simulink model "Furnace"  (R2020a)
settings: Solver=ode15s  StartTime=0  StopTime=27000  FixedStep=0.1  MaxStep=20  MinStep=1e-13  RelTol=1e-08  AbsTol=1e-09
undefined symbols (not defined in the file): agnostic_lqe_params, cont_reg, disturbance_type, F_aI_pid, F_aII_pid, input_type, k, lqe_params, LQR_params, LQRAgnostic_params, MPC_type, MPCDiscrete_function_parameters, MPCDiscreteAgnostic_function_parameters, MPCDiscreteDiffIntegralAgnostic_function_parameters, original_LQR_params, output_type, reg, single_butter_ss
libraries: simulink x35, cstblocks x10, mpclib x3
(part 8 of 8)

== matlab function Furnace/Deprecated, slow loop/Contineous Summer student feedback (Not finished)/Controller/Input  selector2 ==
  data: constant input; signal output; experimental input; controlled input; input_type input
function signal = ChooseSignal(constant, experimental, controlled, input_type)
    switch(input_type)
        case InputType.Experimental
            signal = experimental;
        case InputType.Controlled
            signal = controlled;
        otherwise
            signal = constant;
    end
end

== matlab function Furnace/Deprecated, slow loop/Contineous Summer student feedback (Not finished)/Controller/Input  selector3 ==
  data: constant input; signal output; experimental input; controlled input; input_type input
function signal = ChooseSignal(constant, experimental, controlled, input_type)
    switch(input_type)
        case InputType.Experimental
            signal = experimental;
        case InputType.Controlled
            signal = controlled;
        otherwise
            signal = constant;
    end
end

== matlab function Furnace/Deprecated, slow loop/Contineous Summer student feedback (Not finished)/Controller/Input  selector4 ==
  data: constant input; signal output; experimental input; controlled input; input_type input
function signal = ChooseSignal(constant, experimental, controlled, input_type)
    switch(input_type)
        case InputType.Experimental
            signal = experimental;
        case InputType.Controlled
            signal = controlled;
        otherwise
            signal = constant;
    end
end

== matlab function Furnace/Deprecated, slow loop/Contineous Summer student feedback (Not finished)/Controller/Input  selector5 ==
  data: constant input; signal output; experimental input; controlled input; input_type input
function signal = ChooseSignal(constant, experimental, controlled, input_type)
    switch(input_type)
        case InputType.Experimental
            signal = experimental;
        case InputType.Controlled
            signal = controlled;
        otherwise
            signal = constant;
    end
end

== matlab function Furnace/Deprecated, slow loop/Contineous Summer student feedback (Not finished)/Grate speed/Input selector1 ==
  data: constant input; signal output; experimental input; controlled input; input_type input
function signal = ChooseSignal(constant, experimental, controlled, input_type)
    switch(input_type)
        case InputType.Experimental
            signal = experimental;
        case InputType.Controlled
            signal = controlled;
        otherwise
            signal = constant;
    end
end

== matlab function Furnace/Deprecated, slow loop/Contineous Summer student feedback (Not finished)/Grate speed/Input selector2 ==
  data: constant input; signal output; experimental input; controlled input; input_type input
function signal = ChooseSignal(constant, experimental, controlled, input_type)
    switch(input_type)
        case InputType.Experimental
            signal = experimental;
        case InputType.Controlled
            signal = controlled;
        otherwise
            signal = constant;
    end
end

== matlab function Furnace/Deprecated, slow loop/Contineous Summer student feedback (Not finished)/Secondary air/Input  selector ==
  data: constant input; signal output; experimental input; controlled input; input_type input
function signal = ChooseSignal(constant, experimental, controlled, input_type)
    switch(input_type)
        case InputType.Experimental
            signal = experimental;
        case InputType.Controlled
            signal = controlled;
        otherwise
            signal = constant;
    end
end

== matlab function Furnace/Deprecated, slow loop/Contineous Summer student feedback (Not finished)/Secondary air/Input  selector1 ==
  data: constant input; signal output; experimental input; controlled input; input_type input
function signal = ChooseSignal(constant, experimental, controlled, input_type)
    switch(input_type)
        case InputType.Experimental
            signal = experimental;
        case InputType.Controlled
            signal = controlled;
        otherwise
            signal = constant;
    end
end

== matlab function Furnace/Deprecated, slow loop/Contineous Summer student feedback (Not finished)/Waste and Primary air/Input selector ==
  data: constant input; signal output; experimental input; controlled input; input_type input
function signal = ChooseSignal(constant, experimental, controlled, input_type)
    switch(input_type)
        case InputType.Experimental
            signal = experimental;
        case InputType.Controlled
            signal = controlled;
        otherwise
            signal = constant;
    end
end

== matlab function Furnace/Deprecated, slow loop/Contineous Summer student feedback (Not finished)/Waste and Primary air/Input selector1 ==
  data: constant input; signal output; experimental input; controlled input; input_type input
function signal = ChooseSignal(constant, experimental, controlled, input_type)
    switch(input_type)
        case InputType.Experimental
            signal = experimental;
        case InputType.Controlled
            signal = controlled;
        otherwise
            signal = constant;
    end
end

== matlab function Furnace/Deprecated, slow loop/Contineous Summer student feedback (Not finished)/Waste and Primary air/Input selector2 ==
  data: constant input; signal output; experimental input; controlled input; input_type input
function signal = ChooseSignal(constant, experimental, controlled, input_type)
    switch(input_type)
        case InputType.Experimental
            signal = experimental;
        case InputType.Controlled
            signal = controlled;
        otherwise
            signal = constant;
    end
end

== matlab function Furnace/Deprecated, slow loop/Contineous Summer student feedback (Not finished)/Waste and Primary air/Input selector3 ==
  data: constant input; signal output; experimental input; controlled input; input_type input
function signal = ChooseSignal(constant, experimental, controlled, input_type)
    switch(input_type)
        case InputType.Experimental
            signal = experimental;
        case InputType.Controlled
            signal = controlled;
        otherwise
            signal = constant;
    end
end

== matlab function Furnace/Controller/Controller selector 1 ==
  data: ab input; cascade input; signal output; mpc input; lqr input; controller_type input
function signal = ChooseController(ab, cascade, mpc, lqr,controller_type)
   
switch(controller_type)
        case ControllerType.AB
            signal = ab;
        case ControllerType.Cascade
            signal = cascade;
        case ControllerType.MPC
            signal = mpc;
        otherwise
            signal = lqr;
    end
end

== matlab function Furnace/Controller/Controller selector 2 ==
  data: ab input; cascade input; signal output; mpc input; lqr input; controller_type input
function signal = ChooseController(ab, cascade, mpc, lqr,controller_type)
   
switch(controller_type)
        case ControllerType.AB
            signal = ab;
        case ControllerType.Cascade
            signal = cascade;
        case ControllerType.MPC
            signal = mpc;
        otherwise
            signal = lqr;
    end
end

== matlab function Furnace/Controller/Controller selector 3 ==
  data: ab input; cascade input; signal output; mpc input; lqr input; controller_type input
function signal = ChooseController(ab, cascade, mpc, lqr,controller_type)
   
switch(controller_type)
        case ControllerType.AB
            signal = ab;
        case ControllerType.Cascade
            signal = cascade;
        case ControllerType.MPC
            signal = mpc;
        otherwise
            signal = lqr;
    end
end

== matlab function Furnace/Controller/MPC_subsystem/LQG_controller/Controller_battery/Controller selector 2 ==
  data: MPC_discrete input; MPC_pseudo_discrete input; signal output; LQR input; LQR_diff_integral input; Discrete_MPC_agnostic input; Pseudo_discrete_MPC_agnostic input; LQR_agnostic input; LQR_diff_integral_agnostic input; MPCDiscreteDiffIntegralAgnostic input; MPC_type input
function signal = ChooseMPCType(MPC_discrete,MPC_pseudo_discrete, LQR, LQR_diff_integral,Discrete_MPC_agnostic, Pseudo_discrete_MPC_agnostic, LQR_agnostic, LQR_diff_integral_agnostic, MPCDiscreteDiffIntegralAgnostic, MPC_type)
   
switch(MPC_type)
        % Assuming inputs
        case MPCType.MPCDiscrete
            signal = MPC_discrete;
        case MPCType.MPCPseudoDiscrete
            signal = MPC_pseudo_discrete;
        case MPCType.LQR
            signal = LQR;
        case MPCType.LQRDiffIntegral
            signal = LQR_diff_integral; 
            
        % Agnostic inputs
        case MPCType.MPCDiscreteAgnostic
            signal = Discrete_MPC_agnostic;
        case MPCType.MPCPseudoDiscreteAgnostic
            signal =Pseudo_discrete_MPC_agnostic;
        case MPCType.LQRAgnostic
            signal = LQR_agnostic;
        case MPCType.LQRDiffIntegralAgnostic
            signal = LQR_diff_integral_agnostic; 
    otherwise
        signal = MPCDiscreteDiffIntegralAgnostic; 
    end
end

== matlab function Furnace/Controller/MPC_subsystem/LQG_controller/Controller_battery/MPCDiscrete/MATLAB Function ==
  settings: updateMethod=DISCRETE  sampleTime=MPCDiscrete_params.MPC_plant.Ts
  data: x input; ref input; u_prev input; iA input; u output size=4; MPCDiscrete_function_parameters parameter; new_iA output
function [u, new_iA] = fcn(x, ref, u_prev, iA,...
    MPCDiscrete_function_parameters)


% Discrete_MPC_function_parameter
   % Might just set these manually... 
    MPC_opt = mpcActiveSetOptions;
    MPC_opt.IntegrityChecks = false;
    MPC_opt.UseHessianAsInput = false; 

%% Uncertain part
    new_b0 = MPCDiscrete_function_parameters.b0;
    
    F = (                                           ...
                (MPCDiscrete_function_parameters.F_y_ref* ref)           ...
            +    MPCDiscrete_function_parameters.F_x0*x                  ...
            +    MPCDiscrete_function_parameters.F_du*u_prev    ...
    ); 
% 
    [a,b,c] =mpcActiveSetSolver(                                        ...                    
                                MPCDiscrete_function_parameters.Linv,                        ...                                    
                                F,                                      ...                    
                                MPCDiscrete_function_parameters.Ac,                          ...                                
                                new_b0,                                 ...                        
                                zeros(0,MPCDiscrete_function_parameters.N_prediction_steps), ...                                                        
                                zeros(0,1),                             ...                            
                                iA,                          ...                                
                                MPC_opt                                 ...                        
                            );
    new_iA = double(c); % Overwrite the old iA
    % u = a(1:length(a)/mpc_N_prediction_steps)
%     new_iA = zeros([80,1]); 
%     u = zeros([4,1]); 
    u = a(1:4);

== matlab function Furnace/Controller/MPC_subsystem/LQG_controller/Controller_battery/MPCDiscreteAgnostic/MATLAB Function ==
  settings: updateMethod=DISCRETE  sampleTime=MPCDiscreteAgnostic_params.MPC_plant.Ts
  data: x input; ref input; u_prev input; iA input; u output size=4; MPCDiscreteAgnostic_function_parameters parameter; new_iA output size=size(MPCDiscreteAgnostic_function_parameters.iA)
function [u, new_iA] = fcn(x, ref, u_prev, iA,...
    MPCDiscreteAgnostic_function_parameters)


% Discrete_MPC_function_parameter
   % Might just set these manually... 
    MPC_opt = mpcActiveSetOptions;
    MPC_opt.IntegrityChecks = false;
    MPC_opt.UseHessianAsInput = false; 

%% Uncertain part
    new_b0 = MPCDiscreteAgnostic_function_parameters.b0;
    
    F = (                                           ...
                (MPCDiscreteAgnostic_function_parameters.F_y_ref* ref)           ...
            +    MPCDiscreteAgnostic_function_parameters.F_x0*x                  ...
            +    MPCDiscreteAgnostic_function_parameters.F_du*u_prev    ...
    ); 
% 
    [a,b,c] =mpcActiveSetSolver(                                        ...                    
                                MPCDiscreteAgnostic_function_parameters.Linv,                        ...                                    
                                F,                                      ...                    
                                MPCDiscreteAgnostic_function_parameters.Ac,                          ...                                
                                new_b0,                                 ...                        
                                zeros(0,MPCDiscreteAgnostic_function_parameters.N_prediction_steps), ...                                                        
                                zeros(0,1),                             ...                            
                                iA,                          ...                                
                                MPC_opt                                 ...                        
                            );
    new_iA = double(c); % Overwrite the old iA
    % u = a(1:length(a)/mpc_N_prediction_steps)
%     new_iA = zeros([80,1]); 
%     u = zeros([4,1]); 
    u = a(1:4);

== matlab function Furnace/Controller/MPC_subsystem/LQG_controller/Controller_battery/MPCDiscreteDiffIntegralAgnostic/MATLAB Function ==
  settings: updateMethod=DISCRETE  sampleTime=MPCDiscreteDiffIntegralAgnostic_params.MPC_plant.Ts
  data: x input size=19; ref input; u_prev input; iA input; u output size=4; MPCDiscreteDiffIntegralAgnostic_function_parameters parameter; new_iA output size=size(MPCDiscreteDiffIntegralAgnostic_function_parameters.iA)
function [u, new_iA] = fcn(x, ref, u_prev, iA,...
    MPCDiscreteDiffIntegralAgnostic_function_parameters)


% Discrete_MPC_function_parameter
   % Might just set these manually... 
    MPC_opt = mpcActiveSetOptions;
    MPC_opt.IntegrityChecks = false;
    MPC_opt.UseHessianAsInput = false; 

%% Uncertain part
    new_b0 = MPCDiscreteDiffIntegralAgnostic_function_parameters.b0;
    
    F = (                                           ...
                (MPCDiscreteDiffIntegralAgnostic_function_parameters.F_y_ref* ref)           ...
            +    MPCDiscreteDiffIntegralAgnostic_function_parameters.F_x0*x                  ...
            +    MPCDiscreteDiffIntegralAgnostic_function_parameters.F_du*u_prev    ...
    ); 
% 
    [a,b,c] =mpcActiveSetSolver(                                        ...                    
                                MPCDiscreteDiffIntegralAgnostic_function_parameters.Linv,                        ...                                    
                                F,                                      ...                    
                                MPCDiscreteDiffIntegralAgnostic_function_parameters.Ac,                          ...                                
                                new_b0,                                 ...                        
                                zeros(0,MPCDiscreteDiffIntegralAgnostic_function_parameters.N_prediction_steps), ...                                                        
                                zeros(0,1),                             ...                            
                                iA,                          ...                                
                                MPC_opt                                 ...                        
                            );
    new_iA = double(c); % Overwrite the old iA
    % u = a(1:length(a)/mpc_N_prediction_steps)
%     new_iA = zeros([80,1]); 
%     u = zeros([4,1]); 
    u = a(1:4);

== matlab function Furnace/Actuator dynamics/Waste and Primary air/Input  selector2 ==
  data: constant input; signal output; experimental input; step input; controlled input; input_type input
function signal = ChooseSignal(constant, experimental, step, controlled, input_type)
    switch(input_type)
        case InputType.Experimental
            signal = experimental;
        case InputType.Controlled
            signal = controlled;
        case InputType.Step
            signal = step; 
        otherwise
            signal = constant;
    end
end

== matlab function Furnace/Controller/Controller selector 4 ==
  data: ab input; cascade input; signal output; mpc input; controller_type input
function signal = ChooseController(ab, cascade, mpc,controller_type)
   
switch(controller_type)
        case ControllerType.AB
            signal = ab;
        case ControllerType.Cascade
            signal = cascade;
        otherwise
            signal = mpc;
    end
end

== matlab function Furnace/Controller/MPC_subsystem/LQG_controller/Controller_battery/MPCPseudoDiscrete/Cont mpc ==
  settings: updateMethod=CONTINUOUS  sampleTime=mpc_params.MPC_plant.Ts
  data: u output size=4; x input; ref input size=2; MPCPseudoDiscrete_function_parameters parameter
function u  = fcn(x, ref,...
    MPCPseudoDiscrete_function_parameters)


% Discrete_MPC_function_parameter
   % Might just set these manually... 
    MPC_opt = mpcActiveSetOptions;
    MPC_opt.IntegrityChecks = false;
    MPC_opt.UseHessianAsInput = false; 

%% Uncertain part
    new_b0 = MPCPseudoDiscrete_function_parameters.b0;
    
    F = (                                                                        ...
                (MPCPseudoDiscrete_function_parameters.F_y_ref* ref)           ...
            +    MPCPseudoDiscrete_function_parameters.F_x0*x                  ...
    ); 
% 
    [a,b,c] =mpcActiveSetSolver(                                        ...                    
                                MPCPseudoDiscrete_function_parameters.Linv,                        ...                                    
                                F,                                      ...                    
                                MPCPseudoDiscrete_function_parameters.Ac,                          ...                                
                                new_b0,                                 ...                        
                                zeros(0,MPCPseudoDiscrete_function_parameters.N_prediction_steps), ...                                                        
                                zeros(0,1),                             ...                            
                                zeros(size(new_b0)),                          ...                                
                                MPC_opt                                 ...                        
                            );

%     u = zeros([4,1]); 
    u = a(1:4);

== matlab function Furnace/Controller/MPC_subsystem/LQG_controller/Controller_battery/MPCPseudoDiscreteAgnostic/Cont mpc ==
  settings: updateMethod=CONTINUOUS  sampleTime=mpc_params.MPC_plant.Ts
  data: u output size=4; x input; ref input size=2; MPCPseudoDiscreteAgnostic_function_parameters parameter
function u  = fcn(x, ref,...
    MPCPseudoDiscreteAgnostic_function_parameters)


% Discrete_MPC_function_parameter
   % Might just set these manually... 
    MPC_opt = mpcActiveSetOptions;
    MPC_opt.IntegrityChecks = false;
    MPC_opt.UseHessianAsInput = false; 

%% Uncertain part
    new_b0 = MPCPseudoDiscreteAgnostic_function_parameters.b0;
    
    F = (                                           ...
                (MPCPseudoDiscreteAgnostic_function_parameters.F_y_ref* ref)           ...
            +    MPCPseudoDiscreteAgnostic_function_parameters.F_x0*x                  ...
    ); 
% 
    [a,b,c] =mpcActiveSetSolver(                                        ...                    
                                MPCPseudoDiscreteAgnostic_function_parameters.Linv,                        ...                                    
                                F,                                      ...                    
                                MPCPseudoDiscreteAgnostic_function_parameters.Ac,                          ...                                
                                new_b0,                                 ...                        
                                zeros(0,MPCPseudoDiscreteAgnostic_function_parameters.N_prediction_steps), ...                                                        
                                zeros(0,1),                             ...                            
                                zeros(size(new_b0)),                          ...                                
                                MPC_opt                                 ...                        
                            );

%     u = zeros([4,1]); 
    u = a(1:4);

== matlab function Furnace/Plant2/Boiler/Drum/DIFF_Boiler_vap ==
  data: T_drum input; x_vap output; p input; Mw_water input; M_H2O input; V_EVA input; rho_water input
function x_vap  = Boiler_vap(T_drum,p,Mw_water,M_H2O,V_EVA,rho_water)

R           = 8.314462175*1E3;
%% ENERGY BALANCE EQUATION
x_vap = fzero(@find_x_vap,0);

%%%%%%%%%%%%%%%%%%%%%%%%%%%%%%%%%%%%%%%%%%%%%%%%%%%%%%%%%%%%%%%%%%%%%%%%%%%
    function Res    = find_x_vap(Y)
        x_vap       = Y;
        M_vap       = x_vap.*M_H2O;
        if T_drum < 373.15
            y_sat   = CALC_xsat(T_drum);
            p_vap   = y_sat*p;
            V_vap   = V_EVA - (M_H2O-M_vap)./rho_water;
            Res    = (M_vap-p_vap.*V_vap./(R.*T_drum).*Mw_water);
        else
            [~,T_sat,rho_vap,~,~,~] = SatWater;
            % Density of saturated vapor at T_drum [kg/m3]
            rho_steam   = interp1(T_sat,rho_vap,T_drum,'linear','extrap');
            % Compressibility factor of vapor [-]
            Z_steam     = p.*Mw_water./(rho_steam.*R.*T_drum);
            % Moles of water vapor [kmol]
            N_steam     = M_H2O.*x_vap./Mw_water;
            % Pressure calculated from the vapor fraction [Pa]
            V_steam     = V_EVA-(1-x_vap).*M_H2O./rho_water;
            p2          = Z_steam.*N_steam.*R.*T_drum./V_steam;
            % p2 should be the same as p
            Res         = (p-p2);
        end
    end
end
% function x  = Boiler_vap(T_drum,p,p_amb,Mw_water,V_gas,M_H2O,V_EVA,rho_water)
% 
% R           = 8.314462175*1E3;
% %% ENERGY BALANCE EQUATION
% [p_sat,T_sat,rho_vap,~,~,~] = SatWater;
% x   = fzero(@find_x_vap,0);
% 
% 
% function Res = find_x_vap(Y)
% x_vap   = Y;
% if T_drum < 373.15
%     y_sat   = CALC_xsat(T_drum);
%     p_vap   = y_sat*p_amb;
%     rho_steam = interp1(T_sat,rho_vap,T_drum,'linear','extrap');
%     p_steam = interp1(T_sat,p_sat,T_drum,'linear','extrap');
%     Z_steam = p_steam.*Mw_water./(rho_steam.*R.*T_drum);
%     M_H2O_v = p_vap.*V_gas./(Z_steam.*R.*T_drum).*Mw_water;
%     x_vap2  = M_H2O_v/M_H2O;
%     a       = (x_vap-x_vap2).*1000;
% else
%     rho_steam = interp1(T_sat,rho_vap,T_drum,'linear','extrap');
%     Z_steam = p.*Mw_water./(rho_steam.*R.*T_drum);
%     N_steam = M_H2O.*x_vap./Mw_water;
%     p_vap   = Z_steam.*N_steam.*R.*T_drum./(V_EVA-(1-x_vap).*M_H2O./rho_water);
%     a       = (p-p_vap);
% end
% Res     = a;
% end
% end

== matlab function Furnace/Plant2/Boiler/Economizer/Economizer ==
  data: Fi_fg input; F_w input; Q_ECO output; T_ECO input; T_fg2 input; cp_fg input; epsilon_ECO input; T_fg3 output; eff_HE input; cp_w input; T_ECO2 output
function [Q_ECO,T_fg3,T_ECO2] = CALC_Q_ECO(Fi_fg,F_w,T_ECO,T_fg2,cp_fg,epsilon_ECO,eff_HE, cp_w)

% This function calculates the heat exchanged in the economizer

F_fg    = sum(Fi_fg);
C_min   = cp_fg.*F_fg;
if F_w == 0 
    Q_ECO   = 0;
    T_fg3   = T_fg2;
    T_ECO2  = T_ECO;
else
    Q_ECO   = epsilon_ECO.*C_min.*(T_fg2-T_ECO);
    T_fg3   = T_fg2 - Q_ECO./(cp_fg.*F_fg);
    T_ECO2  = T_ECO + Q_ECO.*eff_HE./(cp_w.*F_w);
end
Q_ECO       = Q_ECO.*eff_HE;

== matlab function Furnace/Plant2/Boiler/Evaporator/Evaporator ==
  data: Fi_fg input; Q_EVA output; T_drum input; T_fg1 input; cp_fg input; epsilon_EVA input; T_fg2 output; eff_HE input
function [Q_EVA, T_fg2] = CALC_Q_EVA(Fi_fg,T_drum,T_fg1,cp_fg,epsilon_EVA,eff_HE)

% This function calculates the heat exchanged in the economizer

F_fg    = sum(Fi_fg);
C_min   = cp_fg.*F_fg;
Q_EVA   = epsilon_EVA.*C_min.*(T_fg1-T_drum);
T_fg2   = T_fg1 - Q_EVA./(cp_fg.*F_fg);
Q_EVA   = Q_EVA.*eff_HE;

== matlab function Furnace/Plant2/Boiler/MATLAB Function ==
  data: p_drum input; k_p_drum input; switch_on output
function switch_on = calc_swch(p_drum, k_p_drum)

switch_on = 0;
if p_drum >= k_p_drum
    switch_on = 1;
end

== matlab function Furnace/Plant2/Boiler/Super heater/Super heater ==
  data: Q_SH output; F_steam input; T_steam output size=1; Fi_fg input; T_drum input; T_fg1 input; cp_fg input; epsilon_SH input; T_fg2 output size=1; eff_HE input
function [Q_SH,T_steam,T_fg2] = CALC_Q_SH(F_steam,Fi_fg,T_drum,T_fg1,cp_fg,epsilon_SH,eff_HE)

% This function calculates the heat exchanged in the super heater

F_fg    = sum(Fi_fg); 

if F_steam == 0 
    T_steam = T_drum;
    T_fg2   = T_fg1;
    Q_SH    = 0;
else
    [~,T_sat,~,~,~,c_p]=SatWater;
    cp_steam= interp1(T_sat,c_p,T_drum,'linear','extrap');
    C_min   = min(cp_fg.*F_fg,cp_steam.*F_steam);
    Q_SH    = epsilon_SH.*C_min.*(T_fg1-T_drum);
    T_fg2   = T_fg1 - Q_SH./(cp_fg.*F_fg);
    T_steam =  T_drum + Q_SH./(cp_steam.*F_steam);
end
Q_SH        = Q_SH.*eff_HE;

== matlab function Furnace/Plant2/Calorific Value/MATLAB Function ==
  data: Fi_fg input; HHV output; T_fg input; cp_fg input; T_amb input; F_aI input; T_aI input; F_aII input; T_aII input
function HHV = CalorificValue(Fi_fg,T_fg,cp_fg,T_amb,F_aI,T_aI,F_aII,T_aII)

HHV = sum(Fi_fg).*cp_fg.*(T_fg-T_amb);%-sum(F_aI).*cp_fg.*(T_aI-T_amb)-F_aII.*cp_fg.*(T_aII-T_amb);

== matlab function Furnace/Plant2/Condenser/District heating heat exchanger ==
  data: F_DH input; Q_HE output; p_HP input; F_turb input; T_return input; cp_water input; epsilon_HE input; Tw_ECO output; T_district output; eff_HE input
function [Q_HE,Tw_ECO,T_district] = CALC_Q_HE(F_DH,p_HP,F_turb,T_return,cp_water,epsilon_HE,eff_HE)

% This function calculates the heat exchanged between the steam from the
% drum and the water from the district heating net
C_min   = cp_water.*F_DH;
[p_sat,T_sat,~,~,~,~] = SatWater;
T_HP    = interp1(p_sat,T_sat,p_HP,'linear','extrap');
if F_turb == 0
    Q_HE    = 0;
else 
    
    Q_HE    = epsilon_HE.*C_min.*(T_HP-T_return);
end
Tw_ECO      = T_HP;
T_district  = T_return + Q_HE./C_min;
Q_HE        = Q_HE./eff_HE;

== matlab function Furnace/Plant2/Flue-gas fan/Fan ==
  data: T_fg input; T_out output; F_fg input; W_el output
function [T_out, W_el] = fcn(T_fg,F_fg)

T_out = T_fg;
W_el = 0;

== matlab function Furnace/Deprecated, slow loop/Furnace/Boiler/Evaporator/Evaporator ==
  data: Fi_fg input; Q_EVA output; T_drum input; T_fg1 input; cp_fg input; epsilon_EVA input; T_fg2 output; eff_HE input
function [Q_EVA, T_fg2] = CALC_Q_EVA(Fi_fg,T_drum,T_fg1,cp_fg,epsilon_EVA,eff_HE)

% This function calculates the heat exchanged in the economizer

F_fg    = sum(Fi_fg);
C_min   = cp_fg.*F_fg;
Q_EVA   = epsilon_EVA.*C_min.*(T_fg1-T_drum);
T_fg2   = T_fg1 - Q_EVA./(cp_fg.*F_fg);
Q_EVA   = Q_EVA.*eff_HE;

== matlab function Furnace/Deprecated, slow loop/Controller/Summer Controller (Cleaned)/Input  selector4 ==
  data: constant input; signal output; experimental input; controlled input; input_type input
function signal = ChooseSignal(constant, experimental, controlled, input_type)
    switch(input_type)
        case InputType.Experimental
            signal = experimental;
        case InputType.Controlled
            signal = controlled;
        otherwise
            signal = constant;
    end
end

== matlab function Furnace/Deprecated, slow loop/Controller/Summer Controller (Cleaned)/Input  selector5 ==
  data: constant input; signal output; experimental input; controlled input; input_type input
function signal = ChooseSignal(constant, experimental, controlled, input_type)
    switch(input_type)
        case InputType.Experimental
            signal = experimental;
        case InputType.Controlled
            signal = controlled;
        otherwise
            signal = constant;
    end
end

== matlab function Furnace/Plant2/Free board/DIFF_Free Board ==
  data: M_fg_int input; dMfg_dt_int output; T_fg input; Fi_in input; T_in input; F_aII input; T_aII input; Q_rad input; p_amb input; dTfg_dt output; Fi_fg_out output; M_fg output; Y_H2O output; V_FreeBoard input; Mw_gas input; T_amb input; cp_fg input; cp_steel input; M_steel_FB input
function [dMfg_dt_int, dTfg_dt,Fi_fg_out,M_fg,Y_H2O] = DIFF_FreeBoard(M_fg_int,T_fg,Fi_in,T_in,F_aII,T_aII,Q_rad,p_amb,V_FreeBoard,Mw_gas,T_amb,cp_fg,cp_steel,M_steel_FB)

% This function calculates the mass and energy balance of the freeboard. The
% furnacefreaboard is treated as one control volume, where the pressure is
% assumed constant in time. 

%%%%%%%%%%%%%%%%%%%%%%%%%%%%%%%%%%%%%%%%%%%%%%%%%%%%%%%%%%%%%%%%%%%%%%%%%%
% Symbol        Units       Explanation
% INPUTS:
% M_fg_int      [kg]        Mass of gas components in the free-board (last
%                           component is missing)
% T_fg          [K]         Temperature flue gas in the free-board
% Fi_in         [kg/s]      Flue gas component mass flows from the grate
% T_in          [K]         Temperature of the flue gas from the grate
% F_aII         [kg/s]      Secondary air mass flow
% T_aII         [K]         Temperature of secondary air 
% Q_rad         [W]         Radiation heat exchanged with the grate
% k              -          Vector of constant parameters
%%%%%%%%%%%%%%%%%%%%%%%%%%%%%%%%%%%%%%%%%%%%%%%%%%%%%%%%%%%%%%%%%%%%%%%%%%

%% Parameters
R           = 8.314462175*1E3;
nc_gas      = size(Fi_in,1);

%%  FLUE GAS  
% Total amount of flue gas in the freeboard is such to have constant p (p=amb)
N_tot       = p_amb.*V_FreeBoard./(R.*T_fg);        % N_tot is used to calculate the amount of the last gas component
N_i         = [M_fg_int./Mw_gas(1:end-1);(N_tot-sum(M_fg_int./Mw_gas(1:end-1)))];  
y_fg        = N_i./N_tot;
Mw_fg       = sum(Mw_gas.*y_fg);
M_fg_tot    = Mw_fg.*N_tot;
M_fg        = N_i.*Mw_gas;
w_fg        = M_fg./M_fg_tot;
Y_H2O       = y_fg(1);

%% INPUTS (functions of time) 
% Gas from grate 
F_in        = sum(Fi_in,1);                         % [kg/s]
w_in        = zeros(size(Fi_in));                   % [kg/kg]
y_in        = zeros(size(Fi_in));
Mw_in       = zeros(size(F_in));
for i = 1:length(F_in)
    w_in(:,i)  = Fi_in(:,i)./F_in(i); 
    y_in(:,i)  = CALC_y_a(w_in(:,i),Mw_gas);        % [kmol/kmol]
    Mw_in(1,i) = sum(Mw_gas.*y_in(:,i));            % [kg/kmol]
end
Q_conv      = sum(F_in.*cp_fg.*(T_in'-T_fg));       % [W]
% Secondary air
w_aII       = CALC_w_ha(T_amb,90,Mw_gas);           % [kg/kg]
Fi_aII      = w_aII.*F_aII;                         % [kg/s]
y_aII       = CALC_y_a(w_aII,Mw_gas);               % [kmol/kmol]
Mw_aII      = sum(Mw_gas.*y_aII);                   % [K]

%% Reaction rates
R_gas       = CALC_Rw_Gas(M_fg,T_fg,nc_gas,Mw_gas,V_FreeBoard);               % [kg/s]
N_gas       = R_gas.R./Mw_gas;                      % [kmol/s]

%% Differential equations
% Temperature equation
dTfg_dt     = 1./(cp_fg.*M_fg_tot+cp_steel.*M_steel_FB).*(Q_conv+F_aII.*cp_fg.*(T_aII-T_fg)+...  	
              R_gas.H+...                                                        
              Q_rad);     
% Time derivative of gas moles in freeboard
dNfg_dt_tot = -N_tot./T_fg.*dTfg_dt;
% Total mole balance
N_out       = sum(F_in./Mw_in) + F_aII./Mw_aII + sum(N_gas) - dNfg_dt_tot;
F_fg_out    = N_out.*Mw_fg;
Fi_fg_out   = F_fg_out.*w_fg;
% Flue gas composition equation
dMfg_dt     = sum(Fi_in,2) + Fi_aII + R_gas.R - Fi_fg_out ;
dMfg_dt_int = dMfg_dt(1:end-1);
